simulink model "projet_CMI_lineaire"  (R2023a)
settings: Solver=VariableStepAuto  StartTime=0.0  StopTime=1  MaxStep=Te/10  RelTol=1e-3
libraries: cstblocks x5
settings Model: Creator=leolebuhotel  LastModifiedBy=leolebuhotel
settings OptimizationCC: ReuseModelBlockBuffer=off

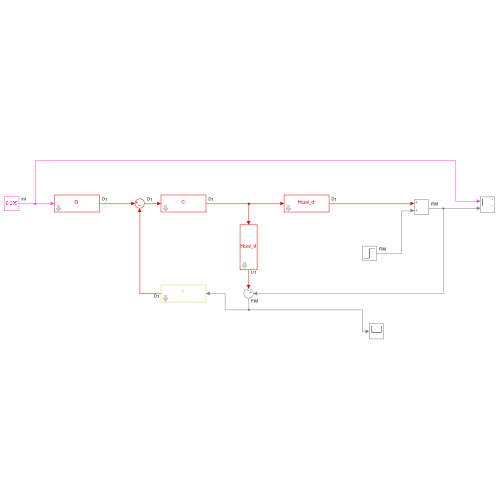
[thumbnail: Simulink's stored preview of the top-level diagram]
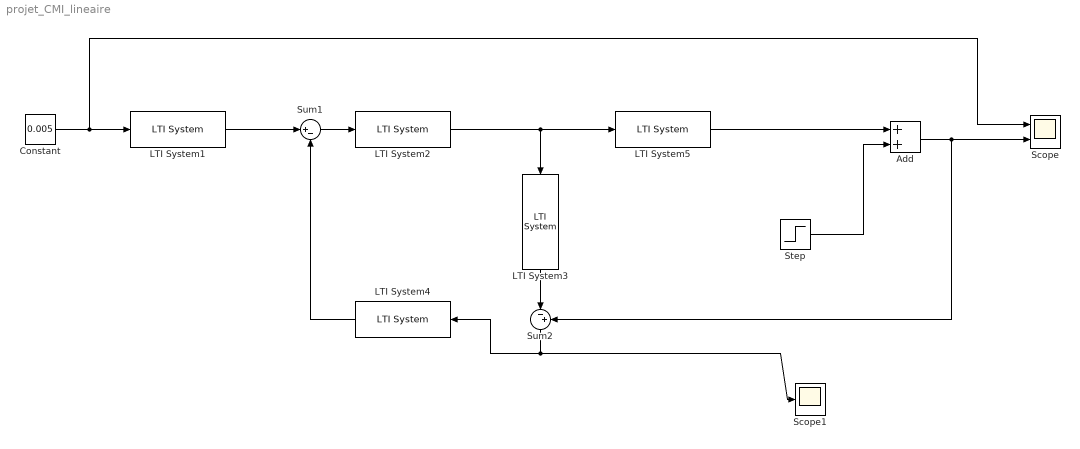
== system projet_CMI_lineaire ==
  Add : Sum
  Constant : Constant  Value=0.005
  LTI System1 : cstblocks/LTI System  sys=G  IC=[]
  LTI System2 : cstblocks/LTI System  sys=C  IC=[]
  LTI System3 : cstblocks/LTI System  sys=Hcmi_d  IC=[]
  LTI System4 : cstblocks/LTI System  sys=F  IC=[]
  LTI System5 : cstblocks/LTI System  sys=Hcmi_d  IC=[]
  Scope : Scope  NumInputPorts=2
  Scope1 : Scope
  Step : Step  Time=0.6  After=0.002  SampleTime=0
  Sum1 : Sum  Inputs=|+-
  Sum2 : Sum  Inputs=|-+
  wires:
  LTI System2/1 -> LTI System5/1, LTI System3/1
  Constant/1 -> Scope/1, LTI System1/1
  Sum1/1 -> LTI System2/1
  LTI System1/1 -> Sum1/1
  LTI System3/1 -> Sum2/1
  Sum2/1 -> Scope1/1, LTI System4/1
  LTI System4/1 -> Sum1/2
  LTI System5/1 -> Add/1
  Add/1 -> Sum2/2, Scope/2
  Step/1 -> Add/2
